simulink model "FunzioneDinamicaInversaSimulink"  (R2020b)
settings: Solver=VariableStepAuto  StartTime=0.0  StopTime=10.0  RelTol=1e-3
undefined symbols (not defined in the file or in its folder): C1_PLV, C2_PLV, theta1ldm, theta1ldm_p, theta2ldm, theta2ldm_p
settings Model: Creator=daniele_ravasio  LastModifiedBy=daniele_ravasio

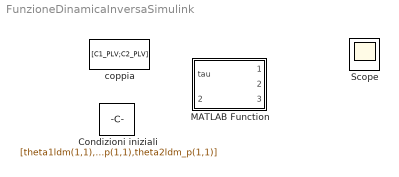
== system FunzioneDinamicaInversaSimulink ==
  Condizioni iniziali : Constant  Value=[theta1ldm(1,1),theta2ldm(1,1),theta1ldm_p(1,1),theta2ldm_p(1,1)]  VectorParams1D=off
  MATLAB Function : MATLAB Function  TreatAsAtomicUnit=on
  Scope : Scope
  coppia : Constant  Value=[C1_PLV;C2_PLV]  VectorParams1D=off

== matlab function FunzioneDinamicaInversaSimulink/MATLAB Function ==
  data: tau input; ThetaInt output; condizioni input; Theta_pInt output; Theta_ppInt output
function  [ThetaInt,Theta_pInt,Theta_ppInt] = fcn(tau,condizioni)

[ThetaInt,Theta_pInt,Theta_ppInt] = DinamicaInversa(tau,condizioni);
end
